simulink subsystem "Inputs_MEGA"  (R2024b)
settings: Solver=VariableStepAuto  StartTime=0.0  StopTime=10.0  RelTol=1e-3
libraries: arduinolib x1
settings Model: Creator=m4ttn  LastModifiedBy=m4ttn

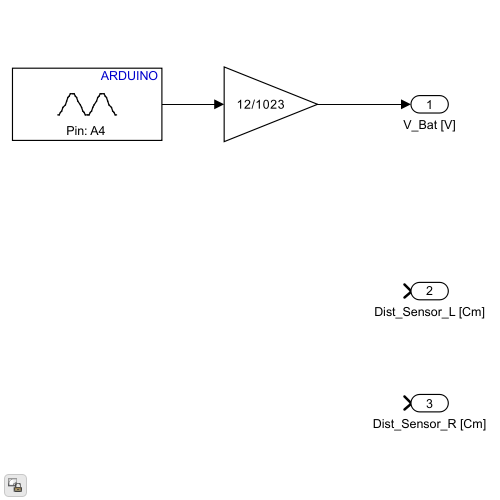
[thumbnail: Simulink's stored preview of the top-level diagram]
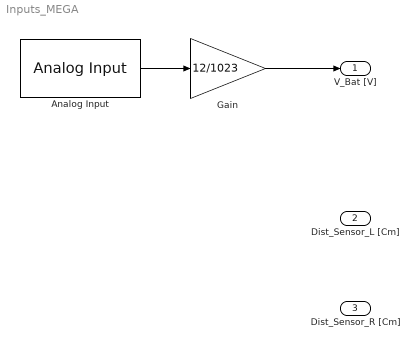
== system Inputs_MEGA ==
  Analog Input : arduinolib/Analog Input  pinNumber=4  ReadResultsOnly=off  ConversionTriggerSource=Software  ExternalTriggerType=uint32( 0 )  OutputDataType=uint16  EnableConversionCompleteNotify=off  EnableOuputStatus=off  SampleTime=-1  blockPlatform=arduino
  Gain : Gain  Gain=12/1023
  V_Bat [V] : Outport
  Dist_Sensor_L [Cm] : Outport  Port=2
  Dist_Sensor_R [Cm] : Outport  Port=3
  wires:
  Analog Input/1 -> Gain/1
  Gain/1 -> V_Bat [V]/1
